simulink model "controller_model"  (R2023b)
settings: Solver=ode3  StartTime=0.0  StopTime=10  RelTol=1e-3
values from neighbouring files (symbols this model uses):
  A = [3.98792656502 1 0 0 0 0 -5.81855146071 0 1 0 0 0 ... (36 elements, 6x6)]    [controller_params.mat]    (also in model_params.mat)
  B = [1 0 0 0 0 0]    [controller_params.mat]    (also in model_params.mat)
  C = [-0.000624151634985 0.000754210232314 -7.15793729404e-05 0 0 0]    [controller_params.mat]    (also in model_params.mat)
  D = 0    [controller_params.mat]    (also in model_params.mat)
  kb = compute_strain_constant('plot_collected_data', true, 'plot_selected_data', true)    [compute_constants.m]    (also in compute_strain_constant.m = P(1); controller_params.mat = -7.77292031464; model_params.mat = -7.77292031464)
  Ki_int = -9.9585416323e-05    [controller_params.mat]    (also in controller_script.m = K_int(n_states+1); controller_script_lab_5.m = K_with_integrator(n_states+1))
  kp = compute_potentiometer_constant('plot_collected_data', true, 'plot_selected_data', true)    [compute_constants.m]    (also in compute_potentiometer_constant.m = P(1); controller_params.mat = 37.3897251534; model_params.mat = 37.3897251534)
  Kx = [0.00571392119727 -0.0170575156897 0.0161429525348 -0.00224203892548 -0.00421804098625 0.00166256586868]    [controller_params.mat]    (also in controller_script_lab_5.m = dlqr(A, B, Q, R))
  Kx_int = [0.00830854997744 -0.0247918532179 0.023451299358 -0.00325101448541 -0.00612843419234 0.00241434428957]    [controller_params.mat]    (also in controller_script.m = K_int(1:n_states); controller_script_lab_5.m = K_with_integrator(1:n_states))
  M = [3543.77501475 3419.31647418 3291.64386704 3161.08265286 3028.02589994 2892.93065581]    [controller_params.mat]    (also in controller_script_lab_5.m = dlqe(A, G, C, Qw, Rv))
  Nbar = 0.0315325549195    [controller_params.mat]    (also in controller_script.m = Nu + Kx*Nx; controller_script_lab_5.m = Nu + Kx*Nx)
  Ts = 0.001    [controller_params.mat]    (also in controller_script.m; controller_script_lab_5.m)
  x_init = [0 0 0 0 0 0]    [controller_params.mat]    (also in controller_script.m = zeros(n_states, 1); controller_script_lab_5.m = zeros(n_states, 1))
undefined symbols (not defined in the file or in its folder): DiscIntNeverNeededParam, MIO, National_Instruments, PCI
libraries: sldrtlib x3
settings Model: SimulationMode=external  ExtModeTrigDuration=30001  Creator=Alunos  LastModifiedBy=olanr
settings SolverCC: AlgebraicLoopSolver=TrustRegion
settings DataIOCC: LimitDataPoints=on  SaveFormat=Array  ReturnWorkspaceOutputs=off
settings OptimizationCC: LifeSpan=inf
settings DebuggingCC: UnconnectedInputMsg=warning  UnconnectedOutputMsg=warning  UnconnectedLineMsg=warning  SFUnexpectedBacktrackingDiag=warning  SFNoUnconditionalDefaultTransitionDiag=warning  SFExecutionAtInitializationDiag=none  ArithmeticOperatorsInVariantConditions=warning
settings HardwareCC: ProdBitPerPointer=32  ProdBitPerSizeT=32  ProdBitPerPtrDiffT=32  ProdLargestAtomicFloat=None  ProdWordSize=32  ProdHWDeviceType=Intel->x86/Pentium  TargetIntDivRoundTo=Zero  TargetEndianess=LittleEndian  TargetHWDeviceType=Intel->x86/Pentium
settings ModelReferenceCC: PropagateSignalLabelsOutOfModel=off
settings SFSimCC: SimUseLocalCustomCode=off  CustomCodeUndefinedFunction=UseInterfaceOnly
settings RTWCC: Description=Simulink Desktop Real-Time  SystemTargetFile=rtwin.tlc  TemplateMakefile=rtwin.tmf  RTWUseLocalCustomCode=off  RTWCompilerOptimization=on
settings CodeAppCC: MaxIdLength=95  StateflowObjectComments=on
settings RTWinTargetCC: TargetPreCompLibLocation=C:\Program Files\MATLAB\R2015a\toolbox\sldrt\lib\win32  MultiwordTypeDef=System defined  DynamicStringBufferSize=256  GroupInternalDataByFunction=off  RemoveDisableFunc=off  RemoveResetFunc=off  MDXCompliant=off  UseToolchainInfoCompliant=off  CoderGroups=[]  AccessMethods=[]  LookupTableObjectStructAxisOrder=1,2,3,4,...  LUTObjectStructOrderExplicitValues=Size,Breakpoints,Table  LUTObjectStructOrderEvenSpacing=Size,Breakpoints,Table  ArrayLayout=Column-major  UnsupportedSFcnMsg=error  ERTHeaderFileRootName=$R$E  ERTSourceFileRootName=$R$E  ERTDataFileRootName=$R_data  OptimizeReductions=off
settings ConfigComp: CovMetricSettings=dw  CovSaveCumulativeToWorkspaceVar=on  CovSaveSingleToWorkspaceVar=on  CovExternalEMLEnable=off

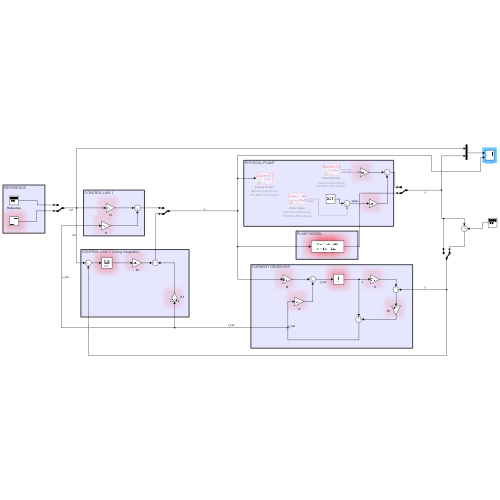
[thumbnail: Simulink's stored preview of the top-level diagram]
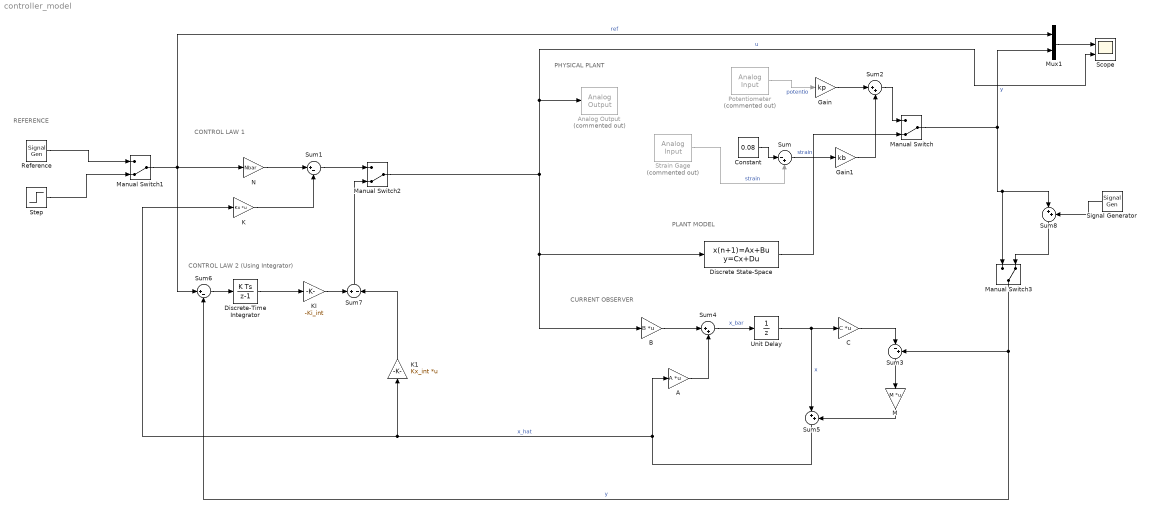
== system controller_model ==
  note: CONTROL LAW 1
  note: REFERENCE
  note: PLANT MODEL
  note: PHYSICAL PLANT
  note: CURRENT OBSERVER
  note: CONTROL LAW 2 (Using Integrator)
  A : Gain  Gain=A  Multiplication=Matrix(K*u)
  Analog Output : sldrtlib/Analog Output  Commented=on  SampleTime=0.001  MaxMissedTicks=10  ShowMissedTicks=off  YieldWhenWaiting=off  DrvName=National_Instruments/PCI-MIO-16E-4  DrvAddress=4294967295  DrvOptions=[0 0 0 0 0 0]  Channels=1  RangeMode=1  VoltRange=1  InitialValue=0  FinalValue=0
      settings: AttributesFormatString=National Instruments\nPCI-MIO-16E-4 [auto]
  B : Gain  Gain=B  Multiplication=Matrix(K*u)
  C : Gain  Gain=C  Multiplication=Matrix(K*u)
  Constant : Constant  Value=0.08
  Discrete State-Space : DiscreteStateSpace  A=A  B=B  C=C  D=D  InitialCondition=x_init  SampleTime=Ts
  Discrete-Time Integrator : DiscreteIntegrator  gainval=1  SampleTime=Ts  ICPrevOutput=DiscIntNeverNeededParam  ICPrevScaledInput=DiscIntNeverNeededParam
  Gain : Gain  Gain=kp
  Gain1 : Gain  Gain=kb
  K : Gain  Gain=Kx  Multiplication=Matrix(K*u)
  K1 : Gain  Gain=Kx_int  Multiplication=Matrix(K*u)
  KI : Gain  Gain=-Ki_int
  M : Gain  Gain=M  Multiplication=Matrix(K*u)
  Manual Switch{,1..3} (4 alike) : ManualSwitch  CurrentSetting=0
  Mux1 : Mux  Inputs=2
  N : Gain  Gain=Nbar
  Potentiometer : sldrtlib/Analog Input  Commented=on  SampleTime=0.001  MaxMissedTicks=10  ShowMissedTicks=off  YieldWhenWaiting=off  DrvName=National_Instruments/PCI-MIO-16E-4  DrvAddress=4294967295  DrvOptions=[0 0 0 0 0 0]  Channels=1  RangeMode=1  VoltRange=1  DataType=1
      settings: AttributesFormatString=National Instruments\nPCI-MIO-16E-4 [auto]
  Reference : SignalGenerator  WaveForm=square  Amplitude=30  Frequency=0.2
  Scope : Scope  NumInputPorts=2
  Signal Generator : SignalGenerator  WaveForm=random  Units=rad/sec
  Step : Step  Time=2  After=30  SampleTime=Ts
  Strain Gage : sldrtlib/Analog Input  Commented=on  SampleTime=0.001  MaxMissedTicks=10  ShowMissedTicks=off  YieldWhenWaiting=off  DrvName=National_Instruments/PCI-MIO-16E-4  DrvAddress=4294967295  DrvOptions=[0 0 0 0 0 0]  Channels=2  RangeMode=1  VoltRange=1  DataType=1
      settings: AttributesFormatString=National Instruments\nPCI-MIO-16E-4 [auto]
  Sum : Sum  Inputs=|-+
  Sum1 : Sum  Inputs=|+-
  Sum{2,4..5,8} (4 alike) : Sum  Inputs=|++
  Sum3 : Sum  Inputs=|-+
  Sum6 : Sum  Inputs=|+-
  Sum7 : Sum  Inputs=+-
  Unit Delay : UnitDelay  InitialCondition=x_init  SampleTime=Ts  HasFrameUpgradeWarning=on
  wires:
  Manual Switch2/1 -> Scope/2, Analog Output/1, B/1, Discrete State-Space/1  "u"
  K/1 -> Sum1/2
  Mux1/1 -> Scope/1
  Potentiometer/1 -> Gain/1  "potentio"
  Sum/1 -> Gain1/1  "strain"
  Constant/1 -> Sum/1
  Gain1/1 -> Sum2/2
  Gain/1 -> Sum2/1
  Strain Gage/1 -> Sum/2  "strain"
  Sum3/1 -> M/1
  Unit Delay/1 -> C/1, Sum5/1  "x"
  Sum4/1 -> Unit Delay/1  "x_bar"
  C/1 -> Sum3/1
  M/1 -> Sum5/2
  A/1 -> Sum4/2
  Sum5/1 -> A/1, K/1, K1/1  "x_hat"
  B/1 -> Sum4/1
  Sum2/1 -> Manual Switch/1
  Discrete State-Space/1 -> Manual Switch/2
  Reference/1 -> Manual Switch1/1
  Manual Switch1/1 -> Sum6/1, Mux1/1, N/1  "ref"
  Step/1 -> Manual Switch1/2
  Manual Switch/1 -> Manual Switch3/1, Sum8/1, Mux1/2  "y"
  Sum6/1 -> Discrete-Time Integrator/1
  N/1 -> Sum1/1
  Sum1/1 -> Manual Switch2/1
  K1/1 -> Sum7/2
  Sum7/1 -> Manual Switch2/2
  Discrete-Time Integrator/1 -> KI/1
  KI/1 -> Sum7/1
  Signal Generator/1 -> Sum8/2
  Sum8/1 -> Manual Switch3/2
  Manual Switch3/1 -> Sum6/2, Sum3/2  "y"
